simulink model "FOODSLIB"  (Simulink 4.00)
settings: Solver=ode5  SolverMode=SingleTasking  StartTime=0.0  StopTime=0  FixedStep=0  MaxStep=0  RelTol=1e-3  AbsTol=1e-6
undefined symbols (not defined in the file or in its folder): comptype, na, tref, turn
(part 1 of 2)
settings Model: SaveTime=off  SaveOutput=off  LimitDataPoints=off  RTWTemplateMakefile=grt_unix.tmf  ExtModeTrigMode=oneshot  ExtModeArmWhenConnect=off  BlockReductionOpt=off

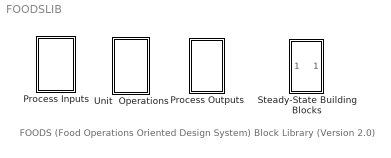
== system FOODSLIB ==
  note: FOODS (Food Operations Oriented Design System) Block Library
      | (Version 2.0)
  Process Inputs : Subsystem
      settings: RTWFcnNameOpts=Auto  RTWFileNameOpts=Auto
  Process Outputs : Subsystem
      settings: RTWFcnNameOpts=Auto  RTWFileNameOpts=Auto
  Steady-State Building Blocks : Subsystem
      settings: RTWFcnNameOpts=Auto  RTWFileNameOpts=Auto
  Unit  Operations : Subsystem
      settings: RTWFcnNameOpts=Auto  RTWFileNameOpts=Auto

== system FOODSLIB/Process Inputs ==
  Air Source : Subsystem
      settings: RTWFcnNameOpts=Auto  RTWFileNameOpts=Auto
      mask Display: plot(0,0,100,100,[80,70,65,60,50,40,35,30,20,80],[60,80,85,90,92,90,85,80,60,60],[48,52,52,48,48],[60,60,34,34,60],[92,8,8,92,92],[55,10,55,10,55])
  Food : Subsystem
      settings: RTWFcnNameOpts=Auto  RTWFileNameOpts=Auto
      mask Display: plot(0,0,100,100,[10,50,50,10,10],[80,80,20,20,80],[50,65,65,50,50],[72,72,28,28,72],[65,80,80,65,65],[64,64,36,36,64])
  Steam Source : Subsystem
      settings: RTWFcnNameOpts=Auto  RTWFileNameOpts=Auto
      mask Display: plot(0,0,100,100,[80,70,65,60,50,40,35,30,20,80],[60,80,85,90,92,90,85,80,60,60],[48,52,52,48,48],[60,60,34,34,60],[92,8,8,92,92],[55,10,55,10,55])
  Steam w/ known Mass Flowrate : Subsystem
      settings: RTWFcnNameOpts=Auto  RTWFileNameOpts=Auto
      mask Display: plot(0,0,100,100,[10,50,50,10,10],[80,80,20,20,80],[50,65,65,50,50],[72,72,28,28,72],[65,80,80,65,65],[64,64,36,36,64])
  Water Source : Subsystem
      settings: RTWFcnNameOpts=Auto  RTWFileNameOpts=Auto
      mask Display: plot(0,0,100,100,[80,70,65,60,50,40,35,30,20,80],[60,80,85,90,92,90,85,80,60,60],[48,52,52,48,48],[60,60,34,34,60],[92,8,8,92,92],[55,10,55,10,55])

== system FOODSLIB/Process Outputs ==
  note: Unconnected Outport (SIMULINK 2.0)
  General No-Cost Output to Workspace : ToWorkspace  VariableName=out  SampleTime=0  SaveFormat=Array
      settings: MaxDataPoints=1
  Product : ToWorkspace  VariableName=out  SampleTime=0  SaveFormat=Array
      settings: MaxDataPoints=1000
  Product with Value : Subsystem
      settings: RTWFcnNameOpts=Auto  RTWFileNameOpts=Auto
  Terminator_2 : Terminator
  Waste : ToWorkspace  VariableName=out  SampleTime=0  SaveFormat=Array
      settings: MaxDataPoints=1000
  Waste with Cost : Subsystem
      settings: RTWFcnNameOpts=Auto  RTWFileNameOpts=Auto
  wires:
  Waste with Cost/1(Outport) -> Waste/1
  Product with Value/1(Outport) -> Product/1

== system FOODSLIB/Steady-State Building Blocks ==
  note: Subset of SIMULINK Block Library (Version 2.0)
  note: Connections:
  note: Function:
  note: Sink:
  note: Source:
  Inport : Inport  Port=1
  Constant : Constant  Value=1
  Demux : Demux  Outputs=3  BusSelectionMode=off
  Mux : Mux  Inputs=3
      settings: DisplayOption=none
  S-Function : S-Function  FunctionName=system  PortCounts=[]  SFunctionModules=''
  To Workspace : ToWorkspace  VariableName=yout  SampleTime=0  SaveFormat=Array
      settings: MaxDataPoints=1000
  Outport : Outport  Port=1

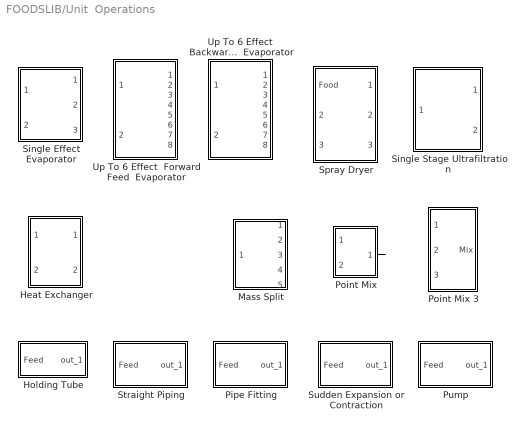
== system FOODSLIB/Unit  Operations ==
  Heat Exchanger : Subsystem
      settings: RTWFcnNameOpts=Auto  RTWFileNameOpts=Auto
  Holding Tube : Subsystem
      settings: RTWFcnNameOpts=Auto  RTWFileNameOpts=Auto
  Mass Split : Subsystem
      settings: RTWFcnNameOpts=Auto  RTWFileNameOpts=Auto
  Pipe Fitting : Subsystem
      settings: RTWFcnNameOpts=Auto  RTWFileNameOpts=Auto
  Point Mix : Subsystem
      settings: RTWFcnNameOpts=Auto  RTWFileNameOpts=Auto
  Point Mix 3 : Subsystem
      settings: RTWFcnNameOpts=Auto  RTWFileNameOpts=Auto
  Pump : Subsystem
      settings: RTWFcnNameOpts=Auto  RTWFileNameOpts=Auto
  Single Effect Evaporator : Subsystem
      settings: RTWFcnNameOpts=Auto  RTWFileNameOpts=Auto
  Single Stage Ultrafiltration : Subsystem
      settings: RTWFcnNameOpts=Auto  RTWFileNameOpts=Auto
  Spray Dryer : Subsystem
      settings: RTWFcnNameOpts=Auto  RTWFileNameOpts=Auto
  Straight Piping : Subsystem
      settings: RTWFcnNameOpts=Auto  RTWFileNameOpts=Auto
  Sudden Expansion or Contraction : Subsystem
      settings: RTWFcnNameOpts=Auto  RTWFileNameOpts=Auto
  Up To 6 Effect  Backward Feed  Evaporator : Subsystem
      settings: RTWFcnNameOpts=Auto  RTWFileNameOpts=Auto
  Up To 6 Effect  Forward Feed  Evaporator : Subsystem
      settings: RTWFcnNameOpts=Auto  RTWFileNameOpts=Auto
  wires:
  Point Mix/1(Mix) -> ?

== system FOODSLIB/Process Inputs/Air Source ==
  Dry Bulb Temperature (C) : Constant  Value=20
  Mux : Mux  Inputs=3
      settings: DisplayOption=none
  Pressure (MPa) : Constant  Value=0.10135
  Relative Humidity (%) : Constant  Value=2.018
  S-Function : S-Function  FunctionName=airs  PortCounts=[]  SFunctionModules=''
  out_1 : Outport  Port=1
  wires:
  Dry Bulb Temperature (C)/1 -> Mux/1
  Pressure (MPa)/1 -> Mux/2
  S-Function/1 -> out_1/1
  Relative Humidity (%)/1 -> Mux/3
  Mux/1 -> S-Function/1

== system FOODSLIB/Process Inputs/Food ==
  Economics Level : Subsystem
      settings: RTWFcnNameOpts=Auto  RTWFileNameOpts=Auto
  Energy Balance Level : Subsystem
      settings: RTWFcnNameOpts=Auto  RTWFileNameOpts=Auto
  Food Quality Kinetics : Subsystem
      settings: RTWFcnNameOpts=Auto  RTWFileNameOpts=Auto
  Food Microbial Death Kinetics : Subsystem
      settings: RTWFcnNameOpts=Auto  RTWFileNameOpts=Auto
  Mass Balance Level : Subsystem
      settings: RTWFcnNameOpts=Auto  RTWFileNameOpts=Auto
  Mux : Mux  Inputs=5
      settings: DisplayOption=none
  S-Function : S-Function  FunctionName=feeds  Parameters='Feed1'  PortCounts=[]  SFunctionModules=''
  out_1 : Outport  Port=1
  wires:
  S-Function/1 -> out_1/1
  Economics Level/1(out_1) -> Mux/5
  Food Quality Kinetics/1(out_1) -> Mux/4
  Food Microbial Death Kinetics/1(out_1) -> Mux/3
  Energy Balance Level/1(out_1) -> Mux/2
  Mass Balance Level/1(out_1) -> Mux/1
  Mux/1 -> S-Function/1

== system FOODSLIB/Process Inputs/Steam Source ==
  Economics Level : Subsystem
      settings: RTWFcnNameOpts=Auto  RTWFileNameOpts=Auto
  Energy Balance Level : Subsystem
      settings: RTWFcnNameOpts=Auto  RTWFileNameOpts=Auto
  More Info : Subsystem
      settings: RTWFcnNameOpts=Auto  RTWFileNameOpts=Auto
      mask Display: disp('?')
  Mux : Mux  Inputs=2
      settings: DisplayOption=none
  S-Function : S-Function  FunctionName=steams  PortCounts=[]  SFunctionModules=''
  out_1 : Outport  Port=1
  wires:
  Mux/1 -> S-Function/1
  Economics Level/1(out_1) -> Mux/2
  Energy Balance Level/1(out_1) -> Mux/1
  S-Function/1 -> out_1/1

== system FOODSLIB/Process Inputs/Steam w/ known Mass Flowrate ==
  Economics Level : Subsystem
      settings: RTWFcnNameOpts=Auto  RTWFileNameOpts=Auto
  Energy Balance Level : Subsystem
      settings: RTWFcnNameOpts=Auto  RTWFileNameOpts=Auto
  Food Quality Kinetics : Subsystem
      settings: RTWFcnNameOpts=Auto  RTWFileNameOpts=Auto
  Food Microbial Death Kinetics : Subsystem
      settings: RTWFcnNameOpts=Auto  RTWFileNameOpts=Auto
  Mass Balance Level : Subsystem
      settings: RTWFcnNameOpts=Auto  RTWFileNameOpts=Auto
  Mux : Mux  Inputs=5
      settings: DisplayOption=none
  S-Function : S-Function  FunctionName=feeds  Parameters='Steam'  PortCounts=[]  SFunctionModules=''
  out_1 : Outport  Port=1
  wires:
  Mux/1 -> S-Function/1
  Mass Balance Level/1(out_1) -> Mux/1
  Energy Balance Level/1(out_1) -> Mux/2
  Food Microbial Death Kinetics/1(out_1) -> Mux/3
  Food Quality Kinetics/1(out_1) -> Mux/4
  Economics Level/1(out_1) -> Mux/5
  S-Function/1 -> out_1/1

== system FOODSLIB/Process Inputs/Water Source ==
  Economics Level : Subsystem
      settings: RTWFcnNameOpts=Auto  RTWFileNameOpts=Auto
  Energy Balance Level : Subsystem
      settings: RTWFcnNameOpts=Auto  RTWFileNameOpts=Auto
  More Info : Subsystem
      settings: RTWFcnNameOpts=Auto  RTWFileNameOpts=Auto
      mask Display: disp('?')
  Mux : Mux  Inputs=2
      settings: DisplayOption=none
  S-Function : S-Function  FunctionName=steams  PortCounts=[]  SFunctionModules=''
  out_1 : Outport  Port=1
  wires:
  Mux/1 -> S-Function/1
  Economics Level/1(out_1) -> Mux/2
  Energy Balance Level/1(out_1) -> Mux/1
  S-Function/1 -> out_1/1

== system FOODSLIB/Process Outputs/Product with Value ==
  in_1 : Inport  Port=1
  Economics Level : Subsystem
      settings: RTWFcnNameOpts=Auto  RTWFileNameOpts=Auto
  Mux : Mux  Inputs=2
      settings: DisplayOption=none
  S-Function : S-Function  FunctionName=products  Parameters='Product1'  PortCounts=[]  SFunctionModules=''
  Outport : Outport  Port=1
  wires:
  Economics Level/1(out_1) -> Mux/2
  S-Function/1 -> Outport/1
  in_1/1 -> Mux/1
  Mux/1 -> S-Function/1

== system FOODSLIB/Process Outputs/Waste with Cost ==
  in_1 : Inport  Port=1
  Economics Level : Subsystem
      settings: RTWFcnNameOpts=Auto  RTWFileNameOpts=Auto
  Mux : Mux  Inputs=2
      settings: DisplayOption=none
  S-Function : S-Function  FunctionName=wastes  Parameters='Waste1'  PortCounts=[]  SFunctionModules=''
  Outport : Outport  Port=1
  wires:
  Economics Level/1(out_1) -> Mux/2
  S-Function/1 -> Outport/1
  in_1/1 -> Mux/1
  Mux/1 -> S-Function/1

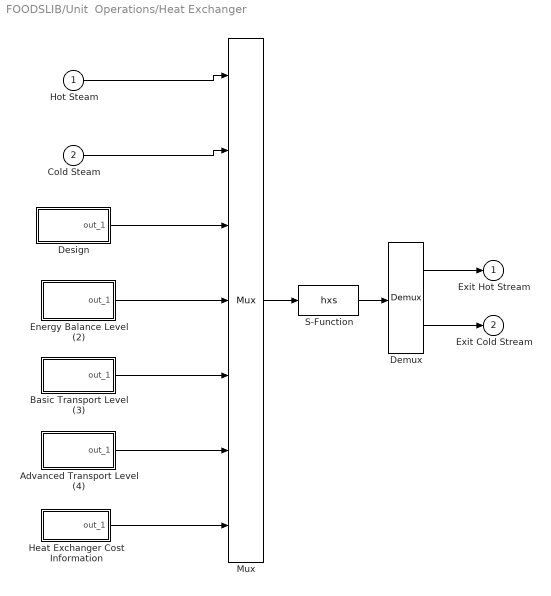
== system FOODSLIB/Unit  Operations/Heat Exchanger ==
  Hot Steam : Inport  Port=1
  Cold Steam : Inport  Port=2
  Advanced Transport Level (4) : Subsystem
      settings: RTWFcnNameOpts=Auto  RTWFileNameOpts=Auto
  Basic Transport Level (3) : Subsystem
      settings: RTWFcnNameOpts=Auto  RTWFileNameOpts=Auto
  Demux : Demux  Outputs=2  BusSelectionMode=off
  Design : Subsystem
      settings: RTWFcnNameOpts=Auto  RTWFileNameOpts=Auto
  Energy Balance Level (2) : Subsystem
      settings: RTWFcnNameOpts=Auto  RTWFileNameOpts=Auto
  Heat Exchanger Cost Information : Subsystem
      settings: RTWFcnNameOpts=Auto  RTWFileNameOpts=Auto
  Mux : Mux  Inputs=7
      settings: DisplayOption=none
  S-Function : S-Function  FunctionName=hxs  Parameters='HX1' 'Steam' '3.5Milk' 'Scond1' 'HotMilk'  PortCounts=[]  SFunctionModules=''
  Exit Hot Stream : Outport  Port=1
  Exit Cold Stream : Outport  Port=2
  wires:
  Hot Steam/1 -> Mux/1
  Cold Steam/1 -> Mux/2
  Mux/1 -> S-Function/1
  Design/1(out_1) -> Mux/3
  Energy Balance Level (2)/1(out_1) -> Mux/4
  Basic Transport Level (3)/1(out_1) -> Mux/5
  Advanced Transport Level (4)/1(out_1) -> Mux/6
  Heat Exchanger Cost Information/1(out_1) -> Mux/7
  Demux/1 -> Exit Hot Stream/1
  Demux/2 -> Exit Cold Stream/1
  S-Function/1 -> Demux/1

== system FOODSLIB/Unit  Operations/Holding Tube ==
  Feed : Inport  Port=1
  Basic Transport Level (3) : Subsystem
      settings: RTWFcnNameOpts=Auto  RTWFileNameOpts=Auto
  Design : Subsystem
      settings: RTWFcnNameOpts=Auto  RTWFileNameOpts=Auto
  Holding Tube Cost Information : Subsystem
      settings: RTWFcnNameOpts=Auto  RTWFileNameOpts=Auto
  Mux1 : Mux  Inputs=4
      settings: DisplayOption=none
  S-Function : S-Function  FunctionName=htbs  Parameters='HoldTube1' 'HotMilk' 'PastMilk'  PortCounts=[]  SFunctionModules=''
  out_1 : Outport  Port=1
  wires:
  Mux1/1 -> S-Function/1
  S-Function/1 -> out_1/1
  Feed/1 -> Mux1/1
  Design/1(out_1) -> Mux1/2
  Basic Transport Level (3)/1(out_1) -> Mux1/3
  Holding Tube Cost Information/1(out_1) -> Mux1/4

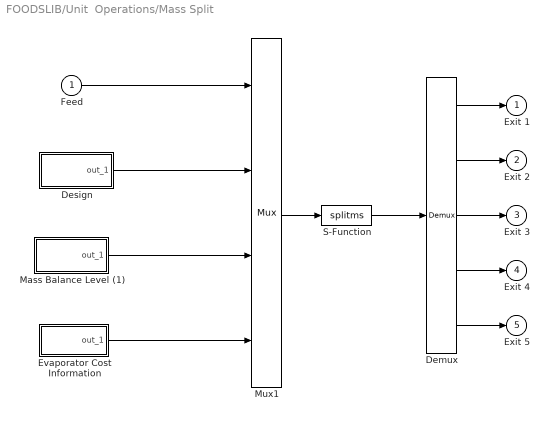
== system FOODSLIB/Unit  Operations/Mass Split ==
  Feed : Inport  Port=1
  Demux : Demux  Outputs=5  BusSelectionMode=off
  Design : Subsystem
      settings: RTWFcnNameOpts=Auto  RTWFileNameOpts=Auto
  Evaporator Cost Information : Subsystem
      settings: RTWFcnNameOpts=Auto  RTWFileNameOpts=Auto
  Mass Balance Level (1) : Subsystem
      settings: RTWFcnNameOpts=Auto  RTWFileNameOpts=Auto
  Mux1 : Mux  Inputs=4
      settings: DisplayOption=none
  S-Function : S-Function  FunctionName=splitms  Parameters='Splitm1' 'Feed' 'Exit1' 'Exit2' 'Exit3' 'Exit4' 'Exit5'  PortCounts=[]  SFunctionModules=''
  Exit 1 : Outport  Port=1
  Exit 2 : Outport  Port=2
  Exit 3 : Outport  Port=3
  Exit 4 : Outport  Port=4
  Exit 5 : Outport  Port=5
  wires:
  Evaporator Cost Information/1(out_1) -> Mux1/4
  Mass Balance Level (1)/1(out_1) -> Mux1/3
  Design/1(out_1) -> Mux1/2
  Demux/5 -> Exit 5/1
  Demux/4 -> Exit 4/1
  Mux1/1 -> S-Function/1
  S-Function/1 -> Demux/1
  Demux/3 -> Exit 3/1
  Demux/2 -> Exit 2/1
  Demux/1 -> Exit 1/1
  Feed/1 -> Mux1/1

== system FOODSLIB/Unit  Operations/Pipe Fitting ==
  Feed : Inport  Port=1
  Advanced Transport Level (4) : Subsystem
      settings: RTWFcnNameOpts=Auto  RTWFileNameOpts=Auto
  Design : Subsystem
      settings: RTWFcnNameOpts=Auto  RTWFileNameOpts=Auto
  Fitting Cost Information : Subsystem
      settings: RTWFcnNameOpts=Auto  RTWFileNameOpts=Auto
  Mux1 : Mux  Inputs=4
      settings: DisplayOption=none
  S-Function : S-Function  FunctionName=fittings  Parameters='Fitting1' 'Feed' 'Exit'  PortCounts=[]  SFunctionModules=''
  out_1 : Outport  Port=1
  wires:
  Fitting Cost Information/1(out_1) -> Mux1/4
  Advanced Transport Level (4)/1(out_1) -> Mux1/3
  Design/1(out_1) -> Mux1/2
  Feed/1 -> Mux1/1
  S-Function/1 -> out_1/1
  Mux1/1 -> S-Function/1

== system FOODSLIB/Unit  Operations/Point Mix ==
  Feed 1 : Inport  Port=1
  Feed 2 : Inport  Port=2
  Design : Subsystem
      settings: RTWFcnNameOpts=Auto  RTWFileNameOpts=Auto
  Mux1 : Mux  Inputs=4
      settings: DisplayOption=none
  Point Mix Cost Information : Subsystem
      settings: RTWFcnNameOpts=Auto  RTWFileNameOpts=Auto
  S-Function : S-Function  FunctionName=mix2s  Parameters='Mix1' 'Feed1' 'Feed2' 'Exit'  PortCounts=[]  SFunctionModules=''
  Mix : Outport  Port=1
  wires:
  Point Mix Cost Information/1(out_1) -> Mux1/4
  Feed 2/1 -> Mux1/2
  Design/1(out_1) -> Mux1/3
  Mux1/1 -> S-Function/1
  S-Function/1 -> Mix/1
  Feed 1/1 -> Mux1/1

== system FOODSLIB/Unit  Operations/Point Mix 3 ==
  Feed 1 : Inport  Port=1
  Feed 2 : Inport  Port=2
  Feed 3 : Inport  Port=3
  Design : Subsystem
      settings: RTWFcnNameOpts=Auto  RTWFileNameOpts=Auto
  Mux1 : Mux  Inputs=5
      settings: DisplayOption=none
  Point Mix Cost Information : Subsystem
      settings: RTWFcnNameOpts=Auto  RTWFileNameOpts=Auto
  S-Function : S-Function  FunctionName=mix3s  Parameters='Mix1' 'Feed1' 'Feed2' 'Feed3' 'Exit'  PortCounts=[]  SFunctionModules=''
  Mix : Outport  Port=1
  wires:
  Feed 1/1 -> Mux1/1
  S-Function/1 -> Mix/1
  Mux1/1 -> S-Function/1
  Feed 2/1 -> Mux1/2
  Feed 3/1 -> Mux1/3
  Design/1(out_1) -> Mux1/4
  Point Mix Cost Information/1(out_1) -> Mux1/5

== system FOODSLIB/Unit  Operations/Pump ==
  Feed : Inport  Port=1
  Basic Transport Level (3) : Subsystem
      settings: RTWFcnNameOpts=Auto  RTWFileNameOpts=Auto
  Design : Subsystem
      settings: RTWFcnNameOpts=Auto  RTWFileNameOpts=Auto
  Mux1 : Mux  Inputs=4
      settings: DisplayOption=none
  Pump Cost Information : Subsystem
      settings: RTWFcnNameOpts=Auto  RTWFileNameOpts=Auto
  S-Function : S-Function  FunctionName=pumps  Parameters='Pump1' 'Feed' 'Exit'  PortCounts=[]  SFunctionModules=''
  out_1 : Outport  Port=1
  wires:
  Pump Cost Information/1(out_1) -> Mux1/4
  Basic Transport Level (3)/1(out_1) -> Mux1/3
  Design/1(out_1) -> Mux1/2
  Feed/1 -> Mux1/1
  S-Function/1 -> out_1/1
  Mux1/1 -> S-Function/1

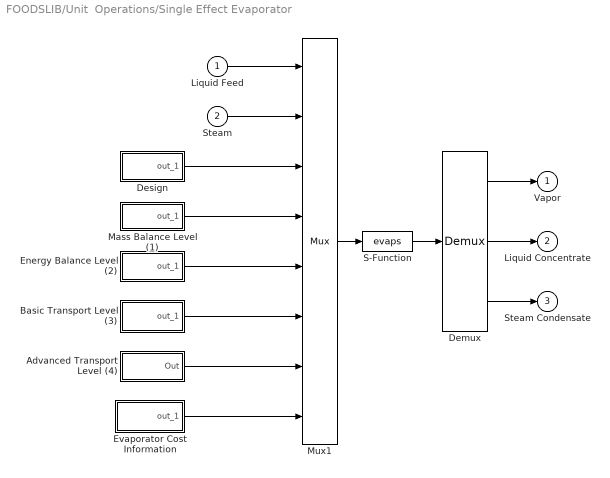
== system FOODSLIB/Unit  Operations/Single Effect Evaporator ==
  Liquid Feed : Inport  Port=1
  Steam : Inport  Port=2
  Advanced Transport Level (4) : Subsystem
      settings: RTWFcnNameOpts=Auto  RTWFileNameOpts=Auto
  Basic Transport Level (3) : Subsystem
      settings: RTWFcnNameOpts=Auto  RTWFileNameOpts=Auto
  Demux : Demux  Outputs=3  BusSelectionMode=off
  Design : Subsystem
      settings: RTWFcnNameOpts=Auto  RTWFileNameOpts=Auto
  Energy Balance Level (2) : Subsystem
      settings: RTWFcnNameOpts=Auto  RTWFileNameOpts=Auto
  Evaporator Cost Information : Subsystem
      settings: RTWFcnNameOpts=Auto  RTWFileNameOpts=Auto
  Mass Balance Level (1) : Subsystem
      settings: RTWFcnNameOpts=Auto  RTWFileNameOpts=Auto
  Mux1 : Mux  Inputs=8
      settings: DisplayOption=none
  S-Function : S-Function  FunctionName=evaps  Parameters='Evap1' 'PastMilk' 'Steam' 'Vapor' 'LiqConc' 'SCond2'  PortCounts=[]  SFunctionModules=''
  Vapor : Outport  Port=1
  Liquid Concentrate : Outport  Port=2
  Steam Condensate : Outport  Port=3
  wires:
  Design/1(out_1) -> Mux1/3
  Mass Balance Level (1)/1(out_1) -> Mux1/4
  Mux1/1 -> S-Function/1
  Steam/1 -> Mux1/2
  Liquid Feed/1 -> Mux1/1
  Energy Balance Level (2)/1(out_1) -> Mux1/5
  Basic Transport Level (3)/1(out_1) -> Mux1/6
  Advanced Transport Level (4)/1(Out) -> Mux1/7
  Evaporator Cost Information/1(out_1) -> Mux1/8
  S-Function/1 -> Demux/1
  Demux/3 -> Steam Condensate/1
  Demux/2 -> Liquid Concentrate/1
  Demux/1 -> Vapor/1

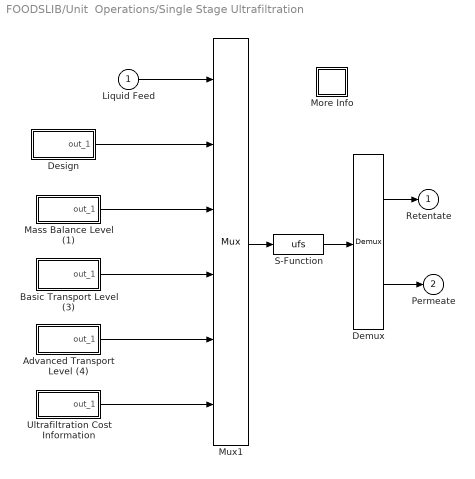
== system FOODSLIB/Unit  Operations/Single Stage Ultrafiltration ==
  Liquid Feed : Inport  Port=1
  Advanced Transport Level (4) : Subsystem
      settings: RTWFcnNameOpts=Auto  RTWFileNameOpts=Auto
  Basic Transport Level (3) : Subsystem
      settings: RTWFcnNameOpts=Auto  RTWFileNameOpts=Auto
  Demux : Demux  Outputs=2  BusSelectionMode=off
  Design : Subsystem
      settings: RTWFcnNameOpts=Auto  RTWFileNameOpts=Auto
  Mass Balance Level (1) : Subsystem
      settings: RTWFcnNameOpts=Auto  RTWFileNameOpts=Auto
  More Info : Subsystem
      settings: RTWFcnNameOpts=Auto  RTWFileNameOpts=Auto
      mask Display: disp('?')
  Mux1 : Mux  Inputs=6
      settings: DisplayOption=none
  S-Function : S-Function  FunctionName=ufs  Parameters='Uf1' 'Feed' 'Retentate' 'Permeate'  PortCounts=[]  SFunctionModules=''
  Ultrafiltration Cost Information : Subsystem
      settings: RTWFcnNameOpts=Auto  RTWFileNameOpts=Auto
  Retentate : Outport  Port=1
  Permeate : Outport  Port=2
  wires:
  Mux1/1 -> S-Function/1
  S-Function/1 -> Demux/1
  Demux/2 -> Permeate/1
  Demux/1 -> Retentate/1
  Liquid Feed/1 -> Mux1/1
  Design/1(out_1) -> Mux1/2
  Mass Balance Level (1)/1(out_1) -> Mux1/3
  Basic Transport Level (3)/1(out_1) -> Mux1/4
  Advanced Transport Level (4)/1(out_1) -> Mux1/5
  Ultrafiltration Cost Information/1(out_1) -> Mux1/6

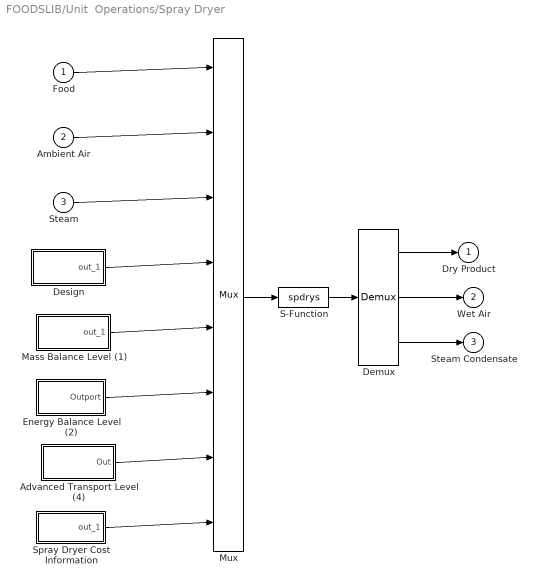
== system FOODSLIB/Unit  Operations/Spray Dryer ==
  Food : Inport  Port=1
  Ambient Air : Inport  Port=2
  Steam : Inport  Port=3
  Advanced Transport Level (4) : Subsystem
      settings: RTWFcnNameOpts=Auto  RTWFileNameOpts=Auto
  Demux : Demux  Outputs=3  BusSelectionMode=off
  Design : Subsystem
      settings: RTWFcnNameOpts=Auto  RTWFileNameOpts=Auto
  Energy Balance Level (2) : Subsystem
      settings: RTWFcnNameOpts=Auto  RTWFileNameOpts=Auto
  Mass Balance Level (1) : Subsystem
      settings: RTWFcnNameOpts=Auto  RTWFileNameOpts=Auto
  Mux : Mux  Inputs=8
      settings: DisplayOption=none
  S-Function : S-Function  FunctionName=spdrys  Parameters='Spdry1' 'LiqConc' 'AmbAir' 'Steam' 'DryMilk' 'WetAir' 'SCond3'  PortCounts=[]  SFunctionModules=''
  Spray Dryer Cost Information : Subsystem
      settings: RTWFcnNameOpts=Auto  RTWFileNameOpts=Auto
  Dry Product : Outport  Port=1
  Wet Air : Outport  Port=2
  Steam Condensate : Outport  Port=3
  wires:
  Food/1 -> Mux/1
  Ambient Air/1 -> Mux/2
  Mux/1 -> S-Function/1
  Steam/1 -> Mux/3
  Design/1(out_1) -> Mux/4
  Mass Balance Level (1)/1(out_1) -> Mux/5
  Energy Balance Level (2)/1(Outport) -> Mux/6
  Advanced Transport Level (4)/1(Out) -> Mux/7
  Spray Dryer Cost Information/1(out_1) -> Mux/8
  Demux/2 -> Wet Air/1
  Demux/1 -> Dry Product/1
  S-Function/1 -> Demux/1
  Demux/3 -> Steam Condensate/1

== system FOODSLIB/Unit  Operations/Straight Piping ==
  Feed : Inport  Port=1
  Advanced Transport Level (4) : Subsystem
      settings: RTWFcnNameOpts=Auto  RTWFileNameOpts=Auto
  Design : Subsystem
      settings: RTWFcnNameOpts=Auto  RTWFileNameOpts=Auto
  Mux1 : Mux  Inputs=4
      settings: DisplayOption=none
  Pipe Cost Information : Subsystem
      settings: RTWFcnNameOpts=Auto  RTWFileNameOpts=Auto
  S-Function : S-Function  FunctionName=pipings  Parameters='Pipe1' 'Feed' 'Exit'  PortCounts=[]  SFunctionModules=''
  out_1 : Outport  Port=1
  wires:
  Mux1/1 -> S-Function/1
  Feed/1 -> Mux1/1
  Design/1(out_1) -> Mux1/2
  Advanced Transport Level (4)/1(out_1) -> Mux1/3
  Pipe Cost Information/1(out_1) -> Mux1/4
  S-Function/1 -> out_1/1

== system FOODSLIB/Unit  Operations/Sudden Expansion or Contraction ==
  Feed : Inport  Port=1
  Advanced Transport Level (4) : Subsystem
      settings: RTWFcnNameOpts=Auto  RTWFileNameOpts=Auto
  Design : Subsystem
      settings: RTWFcnNameOpts=Auto  RTWFileNameOpts=Auto
  Fitting Cost Information : Subsystem
      settings: RTWFcnNameOpts=Auto  RTWFileNameOpts=Auto
  Mux1 : Mux  Inputs=4
      settings: DisplayOption=none
  S-Function : S-Function  FunctionName=sxpcons  Parameters='Fitting1' 'Feed' 'Exit'  PortCounts=[]  SFunctionModules=''
  out_1 : Outport  Port=1
  wires:
  Fitting Cost Information/1(out_1) -> Mux1/4
  Advanced Transport Level (4)/1(out_1) -> Mux1/3
  Design/1(out_1) -> Mux1/2
  Feed/1 -> Mux1/1
  S-Function/1 -> out_1/1
  Mux1/1 -> S-Function/1

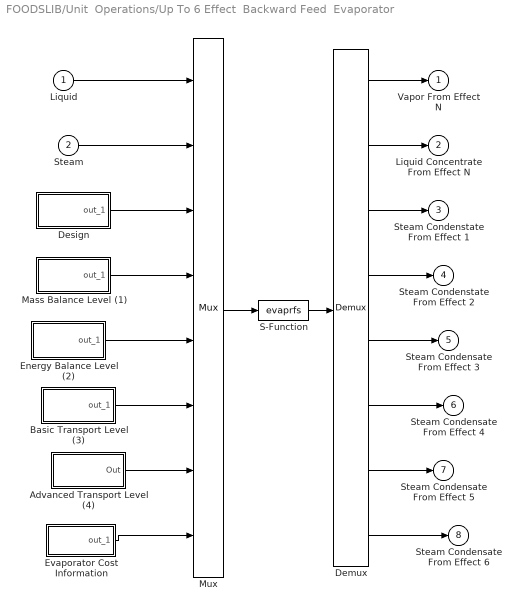
== system FOODSLIB/Unit  Operations/Up To 6 Effect  Backward Feed  Evaporator ==
  Liquid : Inport  Port=1
  Steam : Inport  Port=2
  Advanced Transport Level (4) : Subsystem
      settings: RTWFcnNameOpts=Auto  RTWFileNameOpts=Auto
  Basic Transport Level (3) : Subsystem
      settings: RTWFcnNameOpts=Auto  RTWFileNameOpts=Auto
  Demux : Demux  Outputs=8  BusSelectionMode=off
  Design : Subsystem
      settings: RTWFcnNameOpts=Auto  RTWFileNameOpts=Auto
  Energy Balance Level (2) : Subsystem
      settings: RTWFcnNameOpts=Auto  RTWFileNameOpts=Auto
  Evaporator Cost Information : Subsystem
      settings: RTWFcnNameOpts=Auto  RTWFileNameOpts=Auto
  Mass Balance Level (1) : Subsystem
      settings: RTWFcnNameOpts=Auto  RTWFileNameOpts=Auto
  Mux : Mux  Inputs=8
      settings: DisplayOption=none
  S-Function : S-Function  FunctionName=evaprfs  Parameters='Evap3' 'Feed' 'Steam' 'Vapor' 'Liquid' 'Cond1' 'Cond2' 'Cond3' 'Cond4'  PortCounts=[]  SFunctionModules=''
  Vapor From Effect N : Outport  Port=1
  Liquid Concentrate From Effect N : Outport  Port=2
  Steam Condenstate From Effect 1 : Outport  Port=3
  Steam Condenstate From Effect 2 : Outport  Port=4
  Steam Condensate From Effect 3 : Outport  Port=5
  Steam Condensate From Effect 4 : Outport  Port=6
  Steam Condensate From Effect 5 : Outport  Port=7
  Steam Condensate From Effect 6 : Outport  Port=8
  wires:
  Demux/8 -> Steam Condensate From Effect 6/1
  Demux/7 -> Steam Condensate From Effect 5/1
  Demux/6 -> Steam Condensate From Effect 4/1
  Evaporator Cost Information/1(out_1) -> Mux/8
  Advanced Transport Level (4)/1(Out) -> Mux/7
  Basic Transport Level (3)/1(out_1) -> Mux/6
  Energy Balance Level (2)/1(out_1) -> Mux/5
  Mass Balance Level (1)/1(out_1) -> Mux/4
  Design/1(out_1) -> Mux/3
  Demux/5 -> Steam Condensate From Effect 3/1
  Demux/4 -> Steam Condenstate From Effect 2/1
  Demux/3 -> Steam Condenstate From Effect 1/1
  Demux/2 -> Liquid Concentrate From Effect N/1
  Demux/1 -> Vapor From Effect N/1
  S-Function/1 -> Demux/1
  Mux/1 -> S-Function/1
  Steam/1 -> Mux/2
  Liquid/1 -> Mux/1

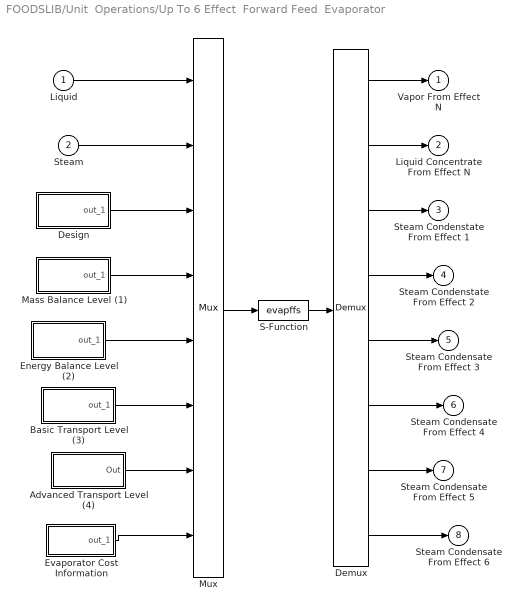
== system FOODSLIB/Unit  Operations/Up To 6 Effect  Forward Feed  Evaporator ==
  Liquid : Inport  Port=1
  Steam : Inport  Port=2
  Advanced Transport Level (4) : Subsystem
      settings: RTWFcnNameOpts=Auto  RTWFileNameOpts=Auto
  Basic Transport Level (3) : Subsystem
      settings: RTWFcnNameOpts=Auto  RTWFileNameOpts=Auto
  Demux : Demux  Outputs=8  BusSelectionMode=off
  Design : Subsystem
      settings: RTWFcnNameOpts=Auto  RTWFileNameOpts=Auto
  Energy Balance Level (2) : Subsystem
      settings: RTWFcnNameOpts=Auto  RTWFileNameOpts=Auto
  Evaporator Cost Information : Subsystem
      settings: RTWFcnNameOpts=Auto  RTWFileNameOpts=Auto
  Mass Balance Level (1) : Subsystem
      settings: RTWFcnNameOpts=Auto  RTWFileNameOpts=Auto
  Mux : Mux  Inputs=8
      settings: DisplayOption=none
  S-Function : S-Function  FunctionName=evapffs  Parameters='Evap3' 'Feed' 'Steam' 'Vapor' 'Liquid' 'Cond1' 'Cond2' 'Cond3' 'Cond4'  PortCounts=[]  SFunctionModules=''
  Vapor From Effect N : Outport  Port=1
  Liquid Concentrate From Effect N : Outport  Port=2
  Steam Condenstate From Effect 1 : Outport  Port=3
  Steam Condenstate From Effect 2 : Outport  Port=4
  Steam Condensate From Effect 3 : Outport  Port=5
  Steam Condensate From Effect 4 : Outport  Port=6
  Steam Condensate From Effect 5 : Outport  Port=7
  Steam Condensate From Effect 6 : Outport  Port=8
  wires:
  Demux/8 -> Steam Condensate From Effect 6/1
  Demux/7 -> Steam Condensate From Effect 5/1
  Demux/6 -> Steam Condensate From Effect 4/1
  Evaporator Cost Information/1(out_1) -> Mux/8
  Advanced Transport Level (4)/1(Out) -> Mux/7
  Basic Transport Level (3)/1(out_1) -> Mux/6
  Energy Balance Level (2)/1(out_1) -> Mux/5
  Mass Balance Level (1)/1(out_1) -> Mux/4
  Design/1(out_1) -> Mux/3
  Demux/5 -> Steam Condensate From Effect 3/1
  Demux/4 -> Steam Condenstate From Effect 2/1
  Demux/3 -> Steam Condenstate From Effect 1/1
  Demux/2 -> Liquid Concentrate From Effect N/1
  Demux/1 -> Vapor From Effect N/1
  S-Function/1 -> Demux/1
  Mux/1 -> S-Function/1
  Steam/1 -> Mux/2
  Liquid/1 -> Mux/1

== system FOODSLIB/Process Inputs/Food/Economics Level ==
  Annual Cost Inflation Rate  (decimal %) : Constant  Value=0.003
  Cost ($/kg) : Constant  Value=0
  Mux1 : Mux  Inputs=2
      settings: DisplayOption=none
  out_1 : Outport  Port=1
  wires:
  Cost ($/kg)/1 -> Mux1/1
  Annual Cost Inflation Rate  (decimal %)/1 -> Mux1/2
  Mux1/1 -> out_1/1

== system FOODSLIB/Process Inputs/Food/Energy Balance Level ==
  Mux1 : Mux  Inputs=3
      settings: DisplayOption=none
  Pressure (MPa) : Constant  Value=0.10135
  Quality (0 - 1) : Constant  Value=na
  Temperature (C) : Constant  Value=20
  out_1 : Outport  Port=1
  wires:
  Mux1/1 -> out_1/1
  Temperature (C)/1 -> Mux1/1
  Pressure (MPa)/1 -> Mux1/2
  Quality (0 - 1)/1 -> Mux1/3

== system FOODSLIB/Process Inputs/Food/Food Quality Kinetics ==
  Activation Energy (kJ/mol) : Constant  Value=100
  D Temperature Base (C) : Constant  Value=121
  D Value (min) : Constant  Value=245
  Mux : Mux  Inputs=5
      settings: DisplayOption=none
  Quality Load : Constant  Value=1
  Z Value (C) : Constant  Value=0
  out_1 : Outport  Port=1
  wires:
  Z Value (C)/1 -> Mux/3
  D Temperature Base (C)/1 -> Mux/2
  D Value (min)/1 -> Mux/1
  Mux/1 -> out_1/1
  Activation Energy (kJ/mol)/1 -> Mux/4
  Quality Load/1 -> Mux/5

== system FOODSLIB/Process Inputs/Food/Food Microbial Death Kinetics ==
  Activation Energy (kJ/mol) : Constant  Value=100
  D Temperature Base (C) : Constant  Value=121
  D Value (min) : Constant  Value=0.02
  Microbial Load : Constant  Value=500000
  Mux : Mux  Inputs=5
      settings: DisplayOption=none
  Z Value (C) : Constant  Value=0
  out_1 : Outport  Port=1
  wires:
  Z Value (C)/1 -> Mux/3
  D Temperature Base (C)/1 -> Mux/2
  D Value (min)/1 -> Mux/1
  Mux/1 -> out_1/1
  Activation Energy (kJ/mol)/1 -> Mux/4
  Microbial Load/1 -> Mux/5

== system FOODSLIB/Process Inputs/Food/Mass Balance Level ==
  Flow Rate (kg/h) : Constant  Value=7200
  Food Composition : Subsystem
      settings: RTWFcnNameOpts=Auto  RTWFileNameOpts=Auto
  Mux1 : Mux  Inputs=2
      settings: DisplayOption=none
  out_1 : Outport  Port=1
  wires:
  Mux1/1 -> out_1/1
  Flow Rate (kg/h)/1 -> Mux1/1
  Food Composition/1(out_1) -> Mux1/2

== system FOODSLIB/Process Inputs/Steam Source/Economics Level ==
  Annual Cost Inflation Rate  (decimal %) : Constant  Value=na
  Cost ($/kg) : Constant  Value=na
  More Info : Subsystem
      settings: RTWFcnNameOpts=Auto  RTWFileNameOpts=Auto
      mask Display: disp('?')
  Mux1 : Mux  Inputs=2
      settings: DisplayOption=none
  out_1 : Outport  Port=1
  wires:
  Cost ($/kg)/1 -> Mux1/1
  Annual Cost Inflation Rate  (decimal %)/1 -> Mux1/2
  Mux1/1 -> out_1/1

== system FOODSLIB/Process Inputs/Steam Source/Energy Balance Level ==
  More Info : Subsystem
      settings: RTWFcnNameOpts=Auto  RTWFileNameOpts=Auto
      mask Display: disp('?')
  Mux : Mux  Inputs=3
      settings: DisplayOption=none
  Quality (0-1) : Constant  Value=1.0
  Temperature (C) : Constant  Value=0
  Vapor Pressure (MPa) : Constant  Value=0.1
  out_1 : Outport  Port=1
  wires:
  Mux/1 -> out_1/1
  Temperature (C)/1 -> Mux/1
  Vapor Pressure (MPa)/1 -> Mux/2
  Quality (0-1)/1 -> Mux/3

== system FOODSLIB/Process Inputs/Steam Source/More Info ==
  note: This block allows a steam source to be defined. The
      | mass flow rate of steam is determined by the demands
      | of the individual unit operations in a given design.

== system FOODSLIB/Process Inputs/Steam w/ known Mass Flowrate/Economics Level ==
  Annual Cost Inflation Rate  (decimal %) : Constant  Value=0.003
  Cost ($/kg) : Constant  Value=0
  Mux1 : Mux  Inputs=2
      settings: DisplayOption=none
  out_1 : Outport  Port=1
  wires:
  Mux1/1 -> out_1/1
  Annual Cost Inflation Rate  (decimal %)/1 -> Mux1/2
  Cost ($/kg)/1 -> Mux1/1

== system FOODSLIB/Process Inputs/Steam w/ known Mass Flowrate/Energy Balance Level ==
  Mux1 : Mux  Inputs=3
      settings: DisplayOption=none
  Pressure (MPa) : Constant  Value=6
  Quality (0 - 1) : Constant  Value=1
  Temperature (C) : Constant  Value=0
  out_1 : Outport  Port=1
  wires:
  Quality (0 - 1)/1 -> Mux1/3
  Pressure (MPa)/1 -> Mux1/2
  Temperature (C)/1 -> Mux1/1
  Mux1/1 -> out_1/1

== system FOODSLIB/Process Inputs/Steam w/ known Mass Flowrate/Food Quality Kinetics ==
  Activation Energy (kJ/mol) : Constant  Value=100
  D Temperature Base (C) : Constant  Value=121
  D Value (min) : Constant  Value=245
  Mux : Mux  Inputs=5
      settings: DisplayOption=none
  Quality Load : Constant  Value=1
  Z Value (C) : Constant  Value=0
  out_1 : Outport  Port=1
  wires:
  Quality Load/1 -> Mux/5
  Activation Energy (kJ/mol)/1 -> Mux/4
  Mux/1 -> out_1/1
  D Value (min)/1 -> Mux/1
  D Temperature Base (C)/1 -> Mux/2
  Z Value (C)/1 -> Mux/3

== system FOODSLIB/Process Inputs/Steam w/ known Mass Flowrate/Food Microbial Death Kinetics ==
  Activation Energy (kJ/mol) : Constant  Value=100
  D Temperature Base (C) : Constant  Value=121
  D Value (min) : Constant  Value=0.02
  Microbial Load : Constant  Value=500000
  Mux : Mux  Inputs=5
      settings: DisplayOption=none
  Z Value (C) : Constant  Value=0
  out_1 : Outport  Port=1
  wires:
  Microbial Load/1 -> Mux/5
  Activation Energy (kJ/mol)/1 -> Mux/4
  Mux/1 -> out_1/1
  D Value (min)/1 -> Mux/1
  D Temperature Base (C)/1 -> Mux/2
  Z Value (C)/1 -> Mux/3

== system FOODSLIB/Process Inputs/Steam w/ known Mass Flowrate/Mass Balance Level ==
  Flow Rate (kg/h) : Constant  Value=10
  Food Composition : Subsystem
      settings: RTWFcnNameOpts=Auto  RTWFileNameOpts=Auto
  Mux1 : Mux  Inputs=2
      settings: DisplayOption=none
  out_1 : Outport  Port=1
  wires:
  Food Composition/1(out_1) -> Mux1/2
  Flow Rate (kg/h)/1 -> Mux1/1
  Mux1/1 -> out_1/1

== system FOODSLIB/Process Inputs/Water Source/Economics Level ==
  Annual Cost Inflation Rate  (decimal %) : Constant  Value=na
  Cost ($/kg) : Constant  Value=na
  More Info : Subsystem
      settings: RTWFcnNameOpts=Auto  RTWFileNameOpts=Auto
      mask Display: disp('?')
  Mux1 : Mux  Inputs=2
      settings: DisplayOption=none
  out_1 : Outport  Port=1
  wires:
  Cost ($/kg)/1 -> Mux1/1
  Annual Cost Inflation Rate  (decimal %)/1 -> Mux1/2
  Mux1/1 -> out_1/1

== system FOODSLIB/Process Inputs/Water Source/Energy Balance Level ==
  More Info : Subsystem
      settings: RTWFcnNameOpts=Auto  RTWFileNameOpts=Auto
      mask Display: disp('?')
  Mux : Mux  Inputs=3
      settings: DisplayOption=none
  Quality (0-1) : Constant  Value=0
  Temperature (C) : Constant  Value=0
  Vapor Pressure (MPa) : Constant  Value=na
  out_1 : Outport  Port=1
  wires:
  Mux/1 -> out_1/1
  Temperature (C)/1 -> Mux/1
  Vapor Pressure (MPa)/1 -> Mux/2
  Quality (0-1)/1 -> Mux/3

== system FOODSLIB/Process Inputs/Water Source/More Info ==
  note: This block allows a water source to be defined. The
      | mass flow rate of water is determined by the demands
      | of the individual unit operations in a given design.

== system FOODSLIB/Process Outputs/Product with Value/Economics Level ==
  Annual Income Inflation Rate (decimal percent) : Constant  Value=0.005
  Income ($/kg) : Constant  Value=1.5
  Mux1 : Mux  Inputs=2
      settings: DisplayOption=none
  out_1 : Outport  Port=1
  wires:
  Mux1/1 -> out_1/1
  Income ($/kg)/1 -> Mux1/1
  Annual Income Inflation Rate (decimal percent)/1 -> Mux1/2

== system FOODSLIB/Process Outputs/Waste with Cost/Economics Level ==
  Annual Cost Inflation Rate (decimal %) : Constant  Value=0.005
  Cost ($/kg) : Constant  Value=1.5
  Mux1 : Mux  Inputs=2
      settings: DisplayOption=none
  out_1 : Outport  Port=1
  wires:
  Mux1/1 -> out_1/1
  Cost ($/kg)/1 -> Mux1/1
  Annual Cost Inflation Rate (decimal %)/1 -> Mux1/2

== system FOODSLIB/Unit  Operations/Heat Exchanger/Advanced Transport Level (4) ==
  Cold Stream  Viscosity Model : Constant  Value=1
  Hot Stream Viscosity Model : Constant  Value=6
  Mux : Mux  Inputs=2
      settings: DisplayOption=none
  out_1 : Outport  Port=1
  wires:
  Hot Stream Viscosity Model/1 -> Mux/1
  Mux/1 -> out_1/1
  Cold Stream  Viscosity Model/1 -> Mux/2

== system FOODSLIB/Unit  Operations/Heat Exchanger/Basic Transport Level (3) ==
  Mux : Mux  Inputs=4
      settings: DisplayOption=none
  Overall Heat Transfer  Coefficient (kJ/h-m^2-K) : Constant  Value=18000
  Plate gap (m) : Constant  Value=0.002
  Plate length  (m) : Constant  Value=0.46
  Plate width (m) : Constant  Value=0.23
  out_1 : Outport  Port=1
  wires:
  Overall Heat Transfer  Coefficient (kJ/h-m^2-K)/1 -> Mux/1
  Mux/1 -> out_1/1
  Plate width (m)/1 -> Mux/2
  Plate gap (m)/1 -> Mux/4
  Plate length  (m)/1 -> Mux/3

== system FOODSLIB/Unit  Operations/Heat Exchanger/Design ==
  Design Level : Constant  Value=4
  Economic Evaluation? : Constant  Value=turn('off')
  Microbial & Quality Assessment? : Constant  Value=turn('off')
  Mux2 : Mux  Inputs=3
      settings: DisplayOption=none
  out_1 : Outport  Port=1
  wires:
  Mux2/1 -> out_1/1
  Design Level/1 -> Mux2/1
  Microbial & Quality Assessment?/1 -> Mux2/2
  Economic Evaluation?/1 -> Mux2/3

== system FOODSLIB/Unit  Operations/Heat Exchanger/Energy Balance Level (2) ==
  Flow Configuration : Constant  Value=1
  Maximum Cold Side Operating Pressure (MPa) : Constant  Value=0.101325
  Maximum Cold Stream Exit Quality ONLY IF WATER/STEAM : Constant  Value=1
  Maximum Cold Stream Exit Temperature (C) : Constant  Value=77
  Minimum Hot Stream Exit Quality ONLY IF WATER/STEAM : Constant  Value=0
  Minimum Hot Stream Exit Temperature (C) : Constant  Value=-tref
  Minimum Temperature  Differential (C) : Constant  Value=10
  More Info : Subsystem
      settings: RTWFcnNameOpts=Auto  RTWFileNameOpts=Auto
      mask Display: disp('?')
  Mux : Mux  Inputs=7
      settings: DisplayOption=none
  out_1 : Outport  Port=1
  wires:
  Flow Configuration/1 -> Mux/1
  Minimum Temperature  Differential (C)/1 -> Mux/2
  Minimum Hot Stream Exit Temperature (C)/1 -> Mux/3
  Mux/1 -> out_1/1
  Maximum Cold Side Operating Pressure (MPa)/1 -> Mux/7
  Maximum Cold Stream Exit Temperature (C)/1 -> Mux/5
  Minimum Hot Stream Exit Quality ONLY IF WATER/STEAM/1 -> Mux/4
  Maximum Cold Stream Exit Quality ONLY IF WATER/STEAM/1 -> Mux/6

== system FOODSLIB/Unit  Operations/Heat Exchanger/Heat Exchanger Cost Information ==
  Base Heat Exchanger Costing Model : Subsystem
      settings: RTWFcnNameOpts=Auto  RTWFileNameOpts=Auto
  Equipment Life (y) : Constant  Value=10
  Maintenance Labor (man-h/h operation) : Constant  Value=0.0075
  Mux : Mux  Inputs=5
      settings: DisplayOption=none
  Operating Labor (man-h/h operation) : Constant  Value=0.125
  Salvage Value  (% of initial cost) : Constant  Value=0.1
  out_1 : Outport  Port=1
  wires:
  Maintenance Labor (man-h/h operation)/1 -> Mux/5
  Operating Labor (man-h/h operation)/1 -> Mux/4
  Equipment Life (y)/1 -> Mux/3
  Salvage Value  (% of initial cost)/1 -> Mux/2
  Base Heat Exchanger Costing Model/1(out_1) -> Mux/1
  Mux/1 -> out_1/1

== system FOODSLIB/Unit  Operations/Holding Tube/Basic Transport Level (3) ==
  Inner Diameter (m) : Constant  Value=0.0525
  Mux : Mux  Inputs=4
      settings: DisplayOption=none
  Number of Log Reductions in N : Constant  Value=15
  Roughness (m) : Constant  Value=0
  Viscosity Model : Constant  Value=1
  out_1 : Outport  Port=1
  wires:
  Inner Diameter (m)/1 -> Mux/1
  Mux/1 -> out_1/1
  Roughness (m)/1 -> Mux/2
  Number of Log Reductions in N/1 -> Mux/3
  Viscosity Model/1 -> Mux/4

== system FOODSLIB/Unit  Operations/Holding Tube/Design ==
  Design Level : Constant  Value=4
  Economic Evaluation? : Constant  Value=turn('off')
  Microbial & Quality Assessment? : Constant  Value=turn('off')
  Mux2 : Mux  Inputs=3
      settings: DisplayOption=none
  out_1 : Outport  Port=1
  wires:
  Mux2/1 -> out_1/1
  Design Level/1 -> Mux2/1
  Microbial & Quality Assessment?/1 -> Mux2/2
  Economic Evaluation?/1 -> Mux2/3

== system FOODSLIB/Unit  Operations/Holding Tube/Holding Tube Cost Information ==
  Base Evaporator Costing Model : Subsystem
      settings: RTWFcnNameOpts=Auto  RTWFileNameOpts=Auto
  Equipment Life (y) : Constant  Value=10
  Maintenance Labor (man-h/h operation) : Constant  Value=0.0075
  Mux : Mux  Inputs=5
      settings: DisplayOption=none
  Operating Labor (man-h/h operation) : Constant  Value=0.125
  Salvage Value  (% of initial cost) : Constant  Value=0.1
  out_1 : Outport  Port=1
  wires:
  Mux/1 -> out_1/1
  Base Evaporator Costing Model/1(out_1) -> Mux/1
  Salvage Value  (% of initial cost)/1 -> Mux/2
  Equipment Life (y)/1 -> Mux/3
  Operating Labor (man-h/h operation)/1 -> Mux/4
  Maintenance Labor (man-h/h operation)/1 -> Mux/5

== system FOODSLIB/Unit  Operations/Mass Split/Design ==
  Design Level : Constant  Value=2
  Economic Evaluation? : Constant  Value=turn('off')
  Microbial & Quality Assessment? : Constant  Value=turn('off')
  Mux2 : Mux  Inputs=3
      settings: DisplayOption=none
  out_1 : Outport  Port=1
  wires:
  Mux2/1 -> out_1/1
  Design Level/1 -> Mux2/1
  Microbial & Quality Assessment?/1 -> Mux2/2
  Economic Evaluation?/1 -> Mux2/3

== system FOODSLIB/Unit  Operations/Mass Split/Evaporator Cost Information ==
  Base Mass Split Costing Model : Subsystem
      settings: RTWFcnNameOpts=Auto  RTWFileNameOpts=Auto
  Equipment Life (y) : Constant  Value=3
  Maintenance Labor (man-h/h operation) : Constant  Value=0.03
  Mux : Mux  Inputs=5
      settings: DisplayOption=none
  Operating Labor (man-h/h operation) : Constant  Value=1
  Salvage Value  (% of initial cost) : Constant  Value=0.1
  out_1 : Outport  Port=1
  wires:
  Maintenance Labor (man-h/h operation)/1 -> Mux/5
  Operating Labor (man-h/h operation)/1 -> Mux/4
  Equipment Life (y)/1 -> Mux/3
  Salvage Value  (% of initial cost)/1 -> Mux/2
  Base Mass Split Costing Model/1(out_1) -> Mux/1
  Mux/1 -> out_1/1

== system FOODSLIB/Unit  Operations/Mass Split/Mass Balance Level (1) ==
  Mass Flow Split  to Exit Stream 1 : Constant  Value=0.25
  Mass Flow Split  to Exit Stream 2 : Constant  Value=0.1
  Mass Flow Split  to Exit Stream 3 : Constant  Value=0
  Mass Flow Split  to Exit Stream 4 : Constant  Value=0
  Mass Flow Split  to Exit Stream 5 : Constant  Value=0
  Mux1 : Mux  Inputs=5
      settings: DisplayOption=none
  out_1 : Outport  Port=1
  wires:
  Mass Flow Split  to Exit Stream 5/1 -> Mux1/5
  Mass Flow Split  to Exit Stream 4/1 -> Mux1/4
  Mass Flow Split  to Exit Stream 3/1 -> Mux1/3
  Mass Flow Split  to Exit Stream 2/1 -> Mux1/2
  Mass Flow Split  to Exit Stream 1/1 -> Mux1/1
  Mux1/1 -> out_1/1

== system FOODSLIB/Unit  Operations/Pipe Fitting/Advanced Transport Level (4) ==
  Diameter (m) : Constant  Value=0.05
  Equivalent Straight Pipe Roughness (m) : Constant  Value=0
  Frictional Loss Coefficient : Constant  Value=0.35
  Mux : Mux  Inputs=4
      settings: DisplayOption=none
  Viscosity Model : Constant  Value=1
  out_1 : Outport  Port=1
  wires:
  Viscosity Model/1 -> Mux/4
  Equivalent Straight Pipe Roughness (m)/1 -> Mux/3
  Frictional Loss Coefficient/1 -> Mux/2
  Diameter (m)/1 -> Mux/1
  Mux/1 -> out_1/1

== system FOODSLIB/Unit  Operations/Pipe Fitting/Design ==
  Design Level : Constant  Value=4
  Economic Evaluation? : Constant  Value=turn('off')
  Microbial & Quality Assessment? : Constant  Value=turn('off')
  Mux2 : Mux  Inputs=3
      settings: DisplayOption=none
  out_1 : Outport  Port=1
  wires:
  Economic Evaluation?/1 -> Mux2/3
  Microbial & Quality Assessment?/1 -> Mux2/2
  Design Level/1 -> Mux2/1
  Mux2/1 -> out_1/1

== system FOODSLIB/Unit  Operations/Pipe Fitting/Fitting Cost Information ==
  Base Evaporator Costing Model : Subsystem
      settings: RTWFcnNameOpts=Auto  RTWFileNameOpts=Auto
  Equipment Life (y) : Constant  Value=3
  Maintenance Labor (man-h/h operation) : Constant  Value=0.03
  Mux : Mux  Inputs=5
      settings: DisplayOption=none
  Operating Labor (man-h/h operation) : Constant  Value=1
  Salvage Value  (% of initial cost) : Constant  Value=0.1
  out_1 : Outport  Port=1
  wires:
  Mux/1 -> out_1/1
  Base Evaporator Costing Model/1(out_1) -> Mux/1
  Salvage Value  (% of initial cost)/1 -> Mux/2
  Equipment Life (y)/1 -> Mux/3
  Operating Labor (man-h/h operation)/1 -> Mux/4
  Maintenance Labor (man-h/h operation)/1 -> Mux/5

== system FOODSLIB/Unit  Operations/Point Mix/Design ==
  Design Level : Constant  Value=2
  Economic Evaluation? : Constant  Value=turn('off')
  Microbial & Quality Assessment? : Constant  Value=turn('off')
  Mux2 : Mux  Inputs=3
      settings: DisplayOption=none
  out_1 : Outport  Port=1
  wires:
  Mux2/1 -> out_1/1
  Design Level/1 -> Mux2/1
  Microbial & Quality Assessment?/1 -> Mux2/2
  Economic Evaluation?/1 -> Mux2/3

== system FOODSLIB/Unit  Operations/Point Mix/Point Mix Cost Information ==
  Base Mass Split Costing Model : Subsystem
      settings: RTWFcnNameOpts=Auto  RTWFileNameOpts=Auto
  Equipment Life (y) : Constant  Value=3
  Maintenance Labor (man-h/h operation) : Constant  Value=0.03
  Mux : Mux  Inputs=5
      settings: DisplayOption=none
  Operating Labor (man-h/h operation) : Constant  Value=1
  Salvage Value  (% of initial cost) : Constant  Value=0.1
  out_1 : Outport  Port=1
  wires:
  Maintenance Labor (man-h/h operation)/1 -> Mux/5
  Operating Labor (man-h/h operation)/1 -> Mux/4
  Equipment Life (y)/1 -> Mux/3
  Salvage Value  (% of initial cost)/1 -> Mux/2
  Base Mass Split Costing Model/1(out_1) -> Mux/1
  Mux/1 -> out_1/1

== system FOODSLIB/Unit  Operations/Point Mix 3/Design ==
  Design Level : Constant  Value=2
  Economic Evaluation? : Constant  Value=turn('off')
  Microbial & Quality Assessment? : Constant  Value=turn('off')
  Mux2 : Mux  Inputs=3
      settings: DisplayOption=none
  out_1 : Outport  Port=1
  wires:
  Economic Evaluation?/1 -> Mux2/3
  Microbial & Quality Assessment?/1 -> Mux2/2
  Design Level/1 -> Mux2/1
  Mux2/1 -> out_1/1

== system FOODSLIB/Unit  Operations/Point Mix 3/Point Mix Cost Information ==
  Base Mass Split Costing Model : Subsystem
      settings: RTWFcnNameOpts=Auto  RTWFileNameOpts=Auto
  Equipment Life (y) : Constant  Value=3
  Maintenance Labor (man-h/h operation) : Constant  Value=0.03
  Mux : Mux  Inputs=5
      settings: DisplayOption=none
  Operating Labor (man-h/h operation) : Constant  Value=1
  Salvage Value  (% of initial cost) : Constant  Value=0.1
  out_1 : Outport  Port=1
  wires:
  Mux/1 -> out_1/1
  Base Mass Split Costing Model/1(out_1) -> Mux/1
  Salvage Value  (% of initial cost)/1 -> Mux/2
  Equipment Life (y)/1 -> Mux/3
  Operating Labor (man-h/h operation)/1 -> Mux/4
  Maintenance Labor (man-h/h operation)/1 -> Mux/5

== system FOODSLIB/Unit  Operations/Pump/Basic Transport Level (3) ==
  Height Differential (m) : Constant  Value=15
  Inlet Diameter (m) : Constant  Value=0.1023
  Motor Efficiency : Constant  Value=1
  Mux : Mux  Inputs=7
      settings: DisplayOption=none
  Outlet Diameter (m) : Constant  Value=0.1023
  Pressure Differential  (MPa) : Constant  Value=6.825e-3
  Pump Efficiency : Constant  Value=0.65
  Viscosity Model : Constant  Value=6
  out_1 : Outport  Port=1
  wires:
  Viscosity Model/1 -> Mux/7
  Motor Efficiency/1 -> Mux/6
  Pump Efficiency/1 -> Mux/5
  Height Differential (m)/1 -> Mux/4
  Pressure Differential  (MPa)/1 -> Mux/3
  Outlet Diameter (m)/1 -> Mux/2
  Inlet Diameter (m)/1 -> Mux/1
  Mux/1 -> out_1/1

== system FOODSLIB/Unit  Operations/Pump/Design ==
  Design Level : Constant  Value=3
  Economic Evaluation? : Constant  Value=turn('off')
  Microbial & Quality Assessment? : Constant  Value=turn('off')
  Mux2 : Mux  Inputs=3
      settings: DisplayOption=none
  out_1 : Outport  Port=1
  wires:
  Economic Evaluation?/1 -> Mux2/3
  Microbial & Quality Assessment?/1 -> Mux2/2
  Design Level/1 -> Mux2/1
  Mux2/1 -> out_1/1

== system FOODSLIB/Unit  Operations/Pump/Pump Cost Information ==
  Base Evaporator Costing Model : Subsystem
      settings: RTWFcnNameOpts=Auto  RTWFileNameOpts=Auto
  Equipment Life (y) : Constant  Value=3
  Maintenance Labor (man-h/h operation) : Constant  Value=0.03
  Mux : Mux  Inputs=5
      settings: DisplayOption=none
  Operating Labor (man-h/h operation) : Constant  Value=1
  Salvage Value  (% of initial cost) : Constant  Value=0.1
  out_1 : Outport  Port=1
  wires:
  Mux/1 -> out_1/1
  Base Evaporator Costing Model/1(out_1) -> Mux/1
  Salvage Value  (% of initial cost)/1 -> Mux/2
  Equipment Life (y)/1 -> Mux/3
  Operating Labor (man-h/h operation)/1 -> Mux/4
  Maintenance Labor (man-h/h operation)/1 -> Mux/5

== system FOODSLIB/Unit  Operations/Single Effect Evaporator/Advanced Transport Level (4) ==
  Evaporator Model Type : Constant  Value=20
  More Info : Subsystem
      settings: RTWFcnNameOpts=Auto  RTWFileNameOpts=Auto
      mask Display: disp('?')
  Mux1 : Mux  Inputs=5
      settings: DisplayOption=none
  Pipe Thermal Conductivity  (kJ/h-m-K) : Constant  Value=162
  Pipe Thickness (m) : Constant  Value=0.00391
  Tube Orientation: Horizontal (0); Vertical (1) : Constant  Value=1
  "Viscosity Model For Product Side " : Constant  Value=1
  Out : Outport  Port=1
  wires:
  Mux1/1 -> Out/1
  Evaporator Model Type/1 -> Mux1/1
  Tube Orientation: Horizontal (0); Vertical (1)/1 -> Mux1/2
  "Viscosity Model For Product Side "/1 -> Mux1/3
  Pipe Thickness (m)/1 -> Mux1/4
  Pipe Thermal Conductivity  (kJ/h-m-K)/1 -> Mux1/5

== system FOODSLIB/Unit  Operations/Single Effect Evaporator/Basic Transport Level (3) ==
  Average fluid velocity per tube (m/s) : Constant  Value=2
  Film thickness (m) : Constant  Value=0.0005
  Inner Pipe Diameter (m) : Constant  Value=0.0525
  Mux1 : Mux  Inputs=4
      settings: DisplayOption=none
  Overall Heat Transfer  Coefficient (kJ/h-m^2-K) : Constant  Value=3600
  out_1 : Outport  Port=1
  wires:
  Film thickness (m)/1 -> Mux1/4
  Mux1/1 -> out_1/1
  Overall Heat Transfer  Coefficient (kJ/h-m^2-K)/1 -> Mux1/1
  Inner Pipe Diameter (m)/1 -> Mux1/2
  Average fluid velocity per tube (m/s)/1 -> Mux1/3

== system FOODSLIB/Unit  Operations/Single Effect Evaporator/Design ==
  Design Level : Constant  Value=4
  Economic Evaluation? : Constant  Value=turn('off')
  Microbial & Quality  Assessment? : Constant  Value=turn('off')
  Mux2 : Mux  Inputs=3
      settings: DisplayOption=none
  out_1 : Outport  Port=1
  wires:
  Mux2/1 -> out_1/1
  Design Level/1 -> Mux2/1
  Microbial & Quality  Assessment?/1 -> Mux2/2
  Economic Evaluation?/1 -> Mux2/3

== system FOODSLIB/Unit  Operations/Single Effect Evaporator/Energy Balance Level (2) ==
  Boiling Point Rise Model : Constant  Value=2
  Exit Steam Quality : Constant  Value=0
  More Info : Subsystem
      settings: RTWFcnNameOpts=Auto  RTWFileNameOpts=Auto
      mask Display: disp('?')
  Mux : Mux  Inputs=3
      settings: DisplayOption=none
  Operating Pressure (MPa) : Constant  Value=0.02
  out_1 : Outport  Port=1
  wires:
  Mux/1 -> out_1/1
  Exit Steam Quality/1 -> Mux/2
  Operating Pressure (MPa)/1 -> Mux/1
  Boiling Point Rise Model/1 -> Mux/3

== system FOODSLIB/Unit  Operations/Single Effect Evaporator/Evaporator Cost Information ==
  Base Evaporator Costing Model : Subsystem
      settings: RTWFcnNameOpts=Auto  RTWFileNameOpts=Auto
  Equipment Life (y) : Constant  Value=10
  Maintenance Labor (man-h/h operation) : Constant  Value=0.015
  Mux : Mux  Inputs=5
      settings: DisplayOption=none
  Operating Labor (man-h/h operation) : Constant  Value=0.25
  Salvage Value  (% of initial cost) : Constant  Value=0.1
  out_1 : Outport  Port=1
  wires:
  Mux/1 -> out_1/1
  Maintenance Labor (man-h/h operation)/1 -> Mux/5
  Operating Labor (man-h/h operation)/1 -> Mux/4
  Equipment Life (y)/1 -> Mux/3
  Salvage Value  (% of initial cost)/1 -> Mux/2
  Base Evaporator Costing Model/1(out_1) -> Mux/1

== system FOODSLIB/Unit  Operations/Single Effect Evaporator/Mass Balance Level (1) ==
  Total Solids of Liquid Concentrate (w/w) : Constant  Value=0.48
  out_1 : Outport  Port=1
  wires:
  Total Solids of Liquid Concentrate (w/w)/1 -> out_1/1
